simulink model "testbench"  (R2025b)
settings: Solver=VariableStepAuto  StartTime=0.0  StopTime=(N+1000)*Ts  RelTol=1e-3
undefined symbols (not defined in the file): Adc, Ain, Fin, OSR
libraries: dspmlti4 x1
settings Model: Creator=brianli  LastModifiedBy=brianli

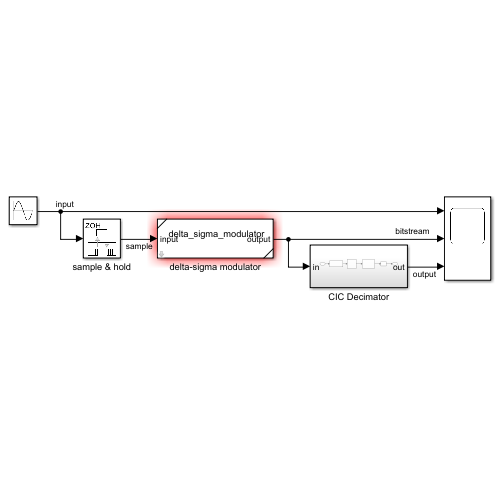
[thumbnail: Simulink's stored preview of the top-level diagram]
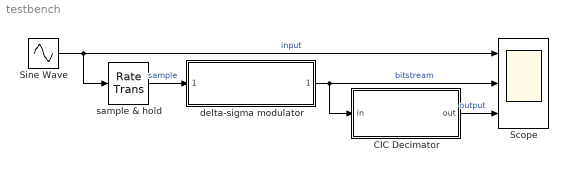
== system testbench ==
  CIC Decimator : Subsystem
  Scope : Scope  NumInputPorts=3
      settings: ActiveDisplayYMinimum=-0.875  ActiveDisplayYMaximum=0.875
  Sine Wave : Sin  Amplitude=Ain  Frequency=2*pi*Fin  SampleTime=0
  delta-sigma modulator : Subsystem  ReferencedSubsystem=delta_sigma_modulator  GBW=GBW  A=Adc
  sample & hold : RateTransition  OutPortSampleTime=Ts
  wires:
  delta-sigma modulator/1 -> CIC Decimator/1(in), Scope/2  "bitstream"
  sample & hold/1 -> delta-sigma modulator/1  "sample"
  Sine Wave/1 -> Scope/1, sample & hold/1  "input"
  CIC Decimator/1(out) -> Scope/3  "output"

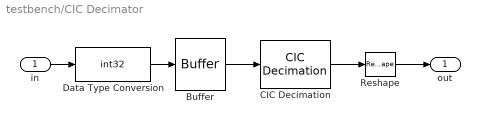
== system testbench/CIC Decimator ==
  in : Inport
  Buffer : Buffer  N=OSR  OutputFrames=off
  CIC Decimation : dspmlti4/CIC Decimation  filtFrom=Dialog parameters  filtobj=CICDECIM  ftype=Decimator  R=OSR  M=1  N=3  filterInternals=Full precision  BPS=[16 16 16 16]  FLPS=0  outputWordLength=32  outputFracLength=0  launchFVT=off  framing=Maintain input frame rate  RateOptions=Enforce single-rate processing
      settings: LibrarySourceBlock=|
      | dsphdlsupportfiltering/CIC
      | Decimation
  Data Type Conversion : DataTypeConversion  OutDataTypeStr=int32  SaturateOnIntegerOverflow=off  RndMeth=Floor
  Reshape : Reshape
  out : Outport
  wires:
  Data Type Conversion/1 -> Buffer/1
  Buffer/1 -> CIC Decimation/1
  in/1 -> Data Type Conversion/1
  Reshape/1 -> out/1
  CIC Decimation/1 -> Reshape/1
